simulink model "costa_loop"  (Simulink 6.6)
settings: Solver=ode45  StartTime=0.0  StopTime=Inf  RelTol=1e-3
undefined symbols (not defined in the file): j
libraries: simulink x3, dspstat3 x3, commsink2 x2, commchan3 x1, commrflib2 x1, commdigbbndpm3 x1, commrandsrc2 x1
settings Model: Creator=master  LastModifiedBy=master

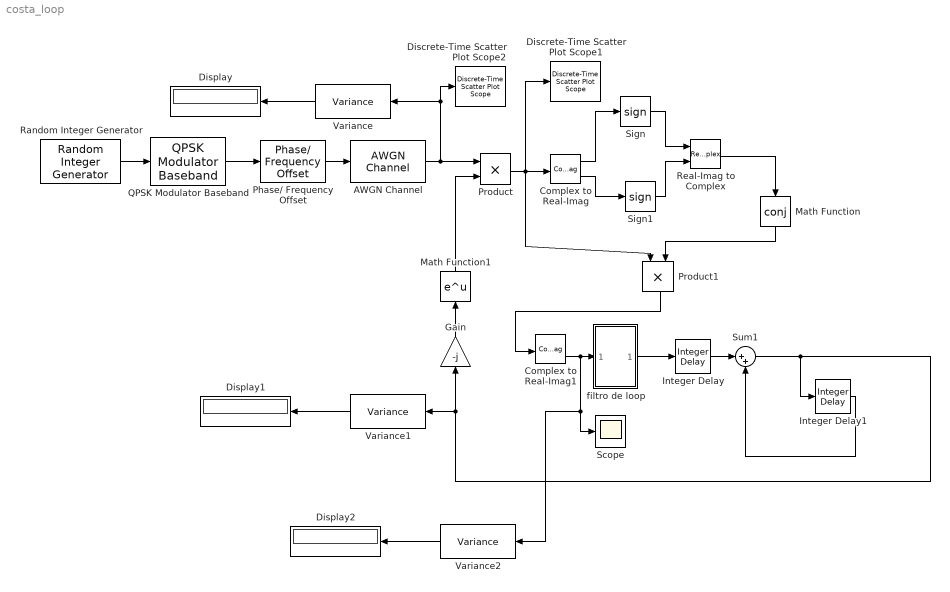
== system costa_loop ==
  AWGN Channel : commchan3/AWGN Channel  SystemSampleTime=-1  seed=67  noiseMode="Signal to noise ratio  (Eb/No)"  EbNodB=30  EsNodB=10  SNRdB=40  bitsPerSym=2  Ps=1  Tsym=1/10000000  variance=1
  Complex to Real-Imag : ComplexToRealImag
  Complex to Real-Imag1 : ComplexToRealImag
  Discrete-Time Scatter Plot Scope1 : commsink2/Discrete-Time Scatter Plot Scope  Tag=ScatterPlot  SystemSampleTime=-1  sampPerSymb=1  offsetEye=0  numTraces=400  numNewFrames=10  LineMarkers=.  LineColors=b  fading=on  render=on  AxisGrid=on  xMin=-0.965127496830596  xMax=0.940552394344232  yMin=-0.948115670330545  yMax=0.957564220844283  inphaseLabel=In-phase Amplitude  quadratureLabel=Quadrature Amplitude  openScopeAtSimStart=on  FrameNumber=off  FigPos=[60 447 400 400]  figTitle=Scatter Plot  numLinesMax=8  block_type_=scatter
  Discrete-Time Scatter Plot Scope2 : commsink2/Discrete-Time Scatter Plot Scope  Tag=ScatterPlot  SystemSampleTime=-1  sampPerSymb=1  offsetEye=0  numTraces=400  numNewFrames=10  LineMarkers=.  LineColors=b  fading=on  render=on  AxisGrid=on  xMin=-1.19064061616857  xMax=1.20200731245399  yMin=-1.17691595732489  yMax=1.21573197129766  inphaseLabel=In-phase Amplitude  quadratureLabel=Quadrature Amplitude  openScopeAtSimStart=on  FrameNumber=off  FigPos=[60 447 400 400]  figTitle=Scatter Plot  numLinesMax=8  block_type_=scatter
  Display : Display
  Display1 : Display
  Display2 : Display
  Gain : Gain  Orientation=up  Gain=-j
  Integer Delay : simulink/Discrete/Integer Delay  vinit=0.0  samptime=-1  NumDelays=1
  Integer Delay1 : simulink/Discrete/Integer Delay  vinit=0.0  samptime=-1  NumDelays=1
  Math Function : Math  Orientation=down  Operator=conj  SaturateOnIntegerOverflow=on
  Math Function1 : Math  Orientation=up  SaturateOnIntegerOverflow=on
  Phase/ Frequency Offset : commrflib2/Phase// Frequency Offset  phaseOffset=30  freqPort=off  freqOffset=0
  Product : Product  RndMeth=Zero
  Product1 : Product  Orientation=down  RndMeth=Zero
  QPSK Modulator Baseband : commdigbbndpm3/QPSK Modulator Baseband  SystemSampleTime=-1  InType=Integer  Enc=Gray  Ph=pi/4  outDtype=double  outWordLen=16  outUDDataType=sfix(16)  outFracLenMode=Best precision  outFracLen=15
  Random Integer Generator : commrandsrc2/Random Integer Generator  SystemSampleTime=-1  mul=4  seed=37  Ts=1/10000000  frameBased=off  sampPerFrame=100  orient=off  outDataType=double
  Real-Imag to Complex : RealImagToComplex
  Scope : Scope
      settings: YMin=-0.01  YMax=0.065
  Sign : Signum
  Sign1 : Signum
  Sum1 : Sum  Inputs=|++
  Variance : dspstat3/Variance  Orientation=left  DialogController=dspDDGCreate  DialogControllerArgs=DataTag0  run=on  reset_popup=None  roundingMode=Floor  overflowMode=off
  Variance1 : dspstat3/Variance  Orientation=left  DialogController=dspDDGCreate  DialogControllerArgs=DataTag1  run=on  reset_popup=None  roundingMode=Floor  overflowMode=off
  Variance2 : dspstat3/Variance  Orientation=left  DialogController=dspDDGCreate  DialogControllerArgs=DataTag2  run=on  reset_popup=None  roundingMode=Floor  overflowMode=off
  filtro de loop : Subsystem
  wires:
  Integer Delay1/1 -> Sum1/2
  Sum1/1 -> Integer Delay1/1, Gain/1, Variance1/1
  filtro de loop/1(Out1) -> Integer Delay/1
  Integer Delay/1 -> Sum1/1
  Random Integer Generator/1 -> QPSK Modulator Baseband/1
  Product/1 -> Complex to Real-Imag/1, Product1/1, Discrete-Time Scatter Plot Scope1/1
  Complex to Real-Imag/1 -> Sign/1
  Complex to Real-Imag/2 -> Sign1/1
  Sign/1 -> Real-Imag to Complex/1
  Sign1/1 -> Real-Imag to Complex/2
  QPSK Modulator Baseband/1 -> Phase/ Frequency Offset/1
  Real-Imag to Complex/1 -> Math Function/1
  Math Function/1 -> Product1/2
  Product1/1 -> Complex to Real-Imag1/1
  Complex to Real-Imag1/2 -> filtro de loop/1(In1), Scope/1, Variance2/1
  Phase/ Frequency Offset/1 -> AWGN Channel/1
  AWGN Channel/1 -> Product/1, Discrete-Time Scatter Plot Scope2/1, Variance/1
  Gain/1 -> Math Function1/1
  Math Function1/1 -> Product/2
  Variance/1 -> Display/1
  Variance1/1 -> Display1/1
  Variance2/1 -> Display2/1

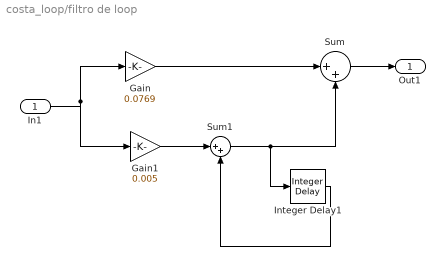
== system costa_loop/filtro de loop ==
  In1 : Inport
  Gain : Gain  Gain=0.0769
  Gain1 : Gain  Gain=0.005
  Integer Delay1 : simulink/Discrete/Integer Delay  vinit=0.0  samptime=-1  NumDelays=1
  Sum : Sum  Inputs=|++
  Sum1 : Sum  Inputs=|++
  Out1 : Outport
  wires:
  Sum/1 -> Out1/1
  In1/1 -> Gain/1, Gain1/1
  Integer Delay1/1 -> Sum1/2
  Sum1/1 -> Sum/2, Integer Delay1/1
  Gain1/1 -> Sum1/1
  Gain/1 -> Sum/1
